simulink model "emergency_scenario"  (R2024b)
settings: Solver=VariableStepAuto  StartTime=0.0  StopTime=simtime  RelTol=1e-3
values from neighbouring files (symbols this model uses):
  m = length(data_p_arrive)    [emergency.m]
undefined symbols (not defined in the file or in its folder): entity, entitySys, get_daparture, n
settings Model: Creator=zahra  LastModifiedBy=zahra

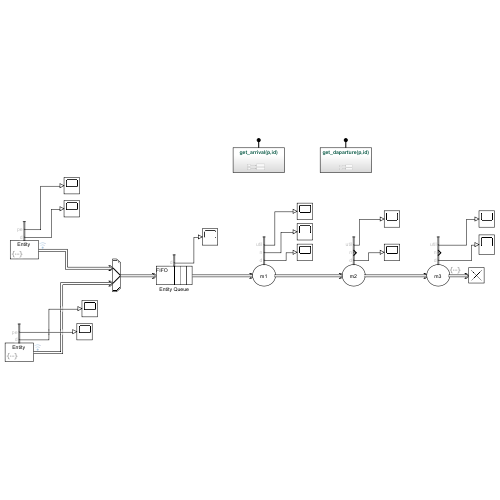
[thumbnail: Simulink's stored preview of the top-level diagram]
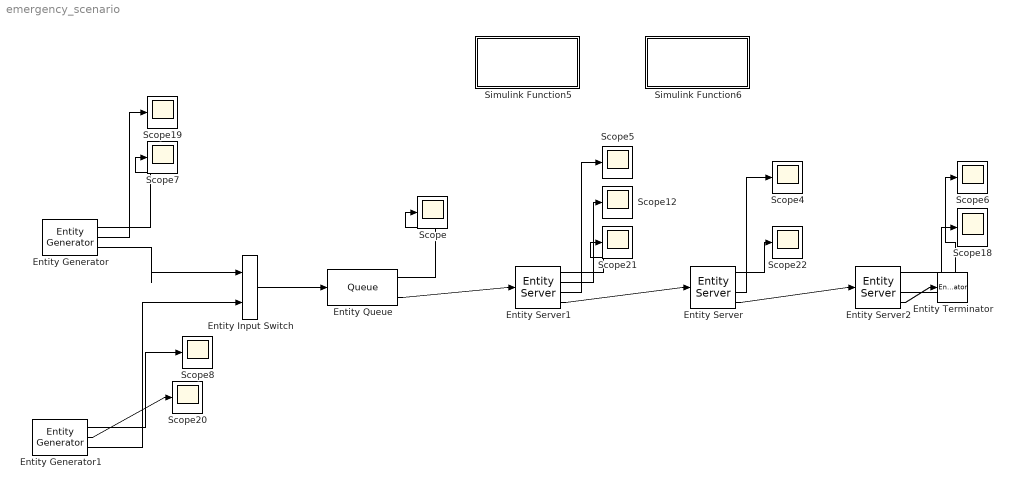
== system emergency_scenario ==
  Entity Input Switch : EntityInputSwitch  InputPortMessageModes=m,m  OutputPortMessageModes=m
  Entity Generator : EntityGenerator  OutputPortMessageModes=n,n,m  TimeSource=MATLAB action  IntergenerationTimeAction=dt=exprnd(1/l_a);  GenerateEntityAtSimulationStart=off  GenerateAction=|  AttributeName=stage1|stage2|stage3|type  AttributeInitialValue=1|2|0.5|1  NumberEntitiesDeparted=on  PendingEntityInBlock=on  EntityType=Structured  EntityTypeName=Entity
      | %rng(123);
      | entity.stage1=exprnd(entity.stage1);
      | entity.stage2=exprnd(entity.stage2);
      | entity.stage3=exprnd(entity.stage3);
      | get_arrival(entitySys.id, entity.type);
      settings: OutputPortMap=o0,o1,o3
  Entity Generator1 : EntityGenerator  OutputPortMessageModes=n,n,m  TimeSource=MATLAB action  IntergenerationTimeAction=dt=exprnd(1/l_t);  GenerateEntityAtSimulationStart=off  GenerateAction=|  AttributeName=stage1|stage2|stage3|type  AttributeInitialValue=0.5|2|1.5|2  NumberEntitiesDeparted=on  PendingEntityInBlock=on  EntityType=Structured  EntityTypeName=Entity
      | %rng(123);
      | entity.stage1=exprnd(entity.stage1);
      | entity.stage2=exprnd(entity.stage2);
      | entity.stage3=exprnd(entity.stage3);
      | get_arrival(entitySys.id, entity.type);
      settings: OutputPortMap=o0,o1,o3
  Entity Queue : Queue  InputPortMessageModes=m  OutputPortMessageModes=n,m  Capacity=Inf  NumberEntitiesDeparted=on
      settings: OutputPortMap=o0,o5
  Entity Server : EntityServer  InputPortMessageModes=m  OutputPortMessageModes=n,n,n,m  Capacity=m2  ServiceTimeSource=Attribute  ServiceTimeAttributeName=stage2  NumberEntitiesDeparted=on  NumberEntitiesInBlock=on  Utilization=on
      settings: OutputPortMap=o0,o1,o5,o9
  Entity Server1 : EntityServer  InputPortMessageModes=m  OutputPortMessageModes=n,n,n,m  Capacity=m1  ServiceTimeSource=Attribute  ServiceTimeAttributeName=stage1  NumberEntitiesDeparted=on  NumberEntitiesInBlock=on  Utilization=on
      settings: OutputPortMap=o0,o1,o5,o9
  Entity Server2 : EntityServer  InputPortMessageModes=m  OutputPortMessageModes=n,n,n,m  Capacity=m3  ServiceTimeSource=Attribute  ServiceTimeAttributeName=stage3  ExitAction=get_daparture(entitySys.id, entity.type);  NumberEntitiesDeparted=on  NumberEntitiesInBlock=on  Utilization=on
      settings: OutputPortMap=o0,o1,o5,o9
  Entity Terminator : EntityTerminator  InputPortMessageModes=m
  Scope{,4..8,12,18..22} (12 alike) : Scope
  Simulink Function5 : Subsystem  TreatAsAtomicUnit=on
  Simulink Function6 : Subsystem  TreatAsAtomicUnit=on
  wires:
  Entity Generator1/3 -> Entity Input Switch/2
  Entity Server2/4 -> Entity Terminator/1
  Entity Server/3 -> Scope4/1
  Entity Server1/3 -> Scope5/1
  Entity Server2/3 -> Scope6/1
  Entity Input Switch/1 -> Entity Queue/1
  Entity Queue/1 -> Scope/1
  Entity Generator/1 -> Scope7/1
  Entity Generator1/1 -> Scope8/1
  Entity Server1/4 -> Entity Server/1
  Entity Server/4 -> Entity Server2/1
  Entity Queue/2 -> Entity Server1/1
  Entity Server1/2 -> Scope12/1
  Entity Generator/3 -> Entity Input Switch/1
  Entity Server2/1 -> Scope18/1
  Entity Generator/2 -> Scope19/1
  Entity Generator1/2 -> Scope20/1
  Entity Server1/1 -> Scope21/1
  Entity Server/1 -> Scope22/1

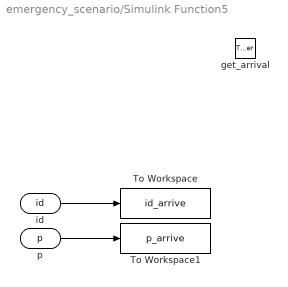
== system emergency_scenario/Simulink Function5 ==
  get_arrival : TriggerPort  TriggerType=function-call  IsSimulinkFunction=on  FunctionName=get_arrival  FunctionVisibility=scoped  VariantControl=(inherit)
  To Workspace : ToWorkspace  VariableName=id_arrive  SaveFormat=Timeseries  SampleTime=-1
  To Workspace1 : ToWorkspace  VariableName=p_arrive  SaveFormat=Timeseries  SampleTime=-1
  p : ArgIn  DisableCoverage=on  ArgumentName=p
  id : ArgIn  DisableCoverage=on  Port=2  ArgumentName=id
  wires:
  p/1 -> To Workspace1/1
  id/1 -> To Workspace/1

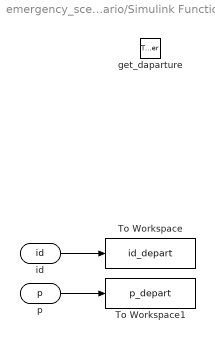
== system emergency_scenario/Simulink Function6 ==
  get_daparture : TriggerPort  TriggerType=function-call  IsSimulinkFunction=on  FunctionName=get_daparture  FunctionVisibility=scoped  VariantControl=(inherit)
  To Workspace : ToWorkspace  VariableName=id_depart  SaveFormat=Timeseries  SampleTime=-1
  To Workspace1 : ToWorkspace  VariableName=p_depart  SaveFormat=Timeseries  SampleTime=-1
  p : ArgIn  DisableCoverage=on  ArgumentName=p
  id : ArgIn  DisableCoverage=on  Port=2  ArgumentName=id
  wires:
  p/1 -> To Workspace1/1
  id/1 -> To Workspace/1
